simulink model "ex_modeling_components"  (R2020a)
settings: Solver=VariableStepAuto  StartTime=0.0  StopTime=10.0  RelTol=1e-3
libraries: simulink x1
settings Model: Creator=The MathWorks, Inc.  LastModifiedBy=Admin
settings DataIOCC: ReturnWorkspaceOutputs=off
settings DebuggingCC: PregeneratedLibrarySubsystemCodeDiagnostic=none  ArithmeticOperatorsInVariantConditions=warning
settings SFSimCC: SimUseLocalCustomCode=off  CustomCodeUndefinedFunction=UseInterfaceOnly
settings RTWCC: RTWUseLocalCustomCode=off

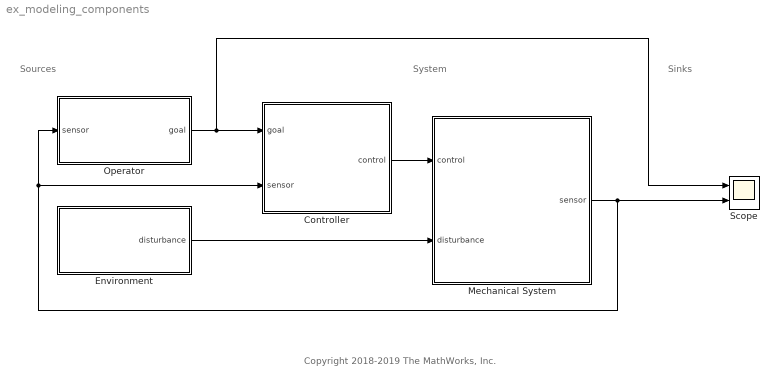
== system ex_modeling_components ==
  note: System
  note: Sources
  note: Copyright 2018-2019 The MathWorks, Inc.
  note: Sinks
  Controller : Subsystem  TreatAsAtomicUnit=on
  Environment : Subsystem
  Mechanical System : Subsystem
  Operator : Subsystem
  Scope : Scope  NumInputPorts=2
  wires:
  Controller/1(control) -> Mechanical System/1(control)
  Mechanical System/1(sensor) -> Operator/1(sensor), Controller/2(sensor), Scope/2
  Environment/1(disturbance) -> Mechanical System/2(disturbance)
  Operator/1(goal) -> Scope/1, Controller/1(goal)

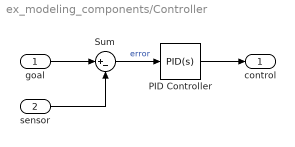
== system ex_modeling_components/Controller ==
  goal : Inport
  sensor : Inport  Port=2
  PID Controller : simulink/Continuous/PID Controller  Controller=PID  Form=Parallel  TimeDomain=Continuous-time  UseExternalTs=off  SampleTime=-1  IntegratorMethod=Forward Euler  FilterMethod=Forward Euler  ControllerParametersSource=internal  P=23.792676457344  I=17.7497318502065  D=7.56800739635058  UseFilter=on  N=49.2376691493838  TunerSelectOption=Transfer Function Based (PID Tuner App)  InitialConditionSource=internal  InitialConditionForIntegrator=0  InitialConditionForFilter=0  DifferentiatorICPrevScaledInput=0  ExternalReset=none  TrackingMode=off  Kt=1  LimitOutput=off  UpperSaturationLimit=inf  LowerSaturationLimit=-inf  LinearizeAsGain=on  AntiWindupMode=none  Kb=1  POutMin=[]  POutMax=[]  IOutMin=[]  IOutMax=[]  DOutMin=[]  DOutMax=[]  NOutMin=[]  NOutMax=[]  SumOutMin=[]  SumOutMax=[]  SaturationOutMin=[]  SaturationOutMax=[]  PParamMin=[]  PParamMax=[]  IParamMin=[]  IParamMax=[]  DParamMin=[]  DParamMax=[]  NParamMin=[]  NParamMax=[]  KbParamMin=[]  KbParamMax=[]  KtParamMin=[]  KtParamMax=[]  KbOutMin=[]  KbOutMax=[]  KtOutMin=[]  KtOutMax=[]  IntegratorOutMin=[]  IntegratorOutMax=[]  FilterOutMin=[]  FilterOutMax=[]  SumI1OutMin=[]  SumI1OutMax=[]  SumI2OutMin=[]  SumI2OutMax=[]  SumI3OutMin=[]  SumI3OutMax=[]  SumI4OutMin=[]  SumI4OutMax=[]  SumDOutMin=[]  SumDOutMax=[]  DifferentiatorOutMin=[]  DifferentiatorOutMax=[]  FilterDiffOutCoefMin=[]  FilterDiffOutCoefMax=[]  ReciprocalOutMin=[]  ReciprocalOutMax=[]  SumDenOutMin=[]  SumDenOutMax=[]  SumNumOutMin=[]  SumNumOutMax=[]  DivideOutMin=[]  DivideOutMax=[]  UdiffTsProdOutMin=[]  UdiffTsProdOutMax=[]  NTsProdOutMin=[]  NTsProdOutMax=[]  UintegralTsProdOutMin=[]  UintegralTsProdOutMax=[]  UngainTsProdOutMin=[]  UngainTsProdOutMax=[]  IntegratorContinuousStateAttributes=''  IntegratorStateMustResolveToSignalObject=off  IntegratorRTWStateStorageClass=Auto  FilterContinuousStateAttributes=''  FilterStateMustResolveToSignalObject=off  FilterRTWStateStorageClass=Auto  ParallelPVariant=InternalParameters  IdealPVariant=Disabled  IVariant=InternalParameters  DVariant=InternalParameters  IntegratorVariant=Continuous  SatVariant=Disabled  AWVariant=Passthrough  PCopyVariant=Disabled  TRVariant=Disabled  FdbkBlocksVariant=Forward  IdealPFdbkVariant=Disabled  SatFdbkVariant=Disabled  DerivativeFilterVariant=ContFilter  NVariant=InternalParameters  NCopyVariant=Disabled  FilterICVariant=InternalICsFilter  IntegratorICVariant=InternalICs  ExternalResetVariant=Disabled  TRSumVariant=Passthrough  SumFdbkVariant=Disabled  SumVariant=Sum_PID  TsampFilterVariant=InternalTs  TsampNgainVariant=Passthrough  TsampIntegralVariant=Passthrough
  Sum : Sum  Inputs=|+-
  control : Outport  VectorParamsAs1DForOutWhenUnconnected=off
  wires:
  goal/1 -> Sum/1
  Sum/1 -> PID Controller/1  "error"
  PID Controller/1 -> control/1
  sensor/1 -> Sum/2

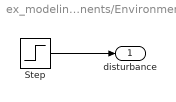
== system ex_modeling_components/Environment ==
  Step : Step  Time=5  After=10  SampleTime=0
  disturbance : Outport  VectorParamsAs1DForOutWhenUnconnected=off
  wires:
  Step/1 -> disturbance/1

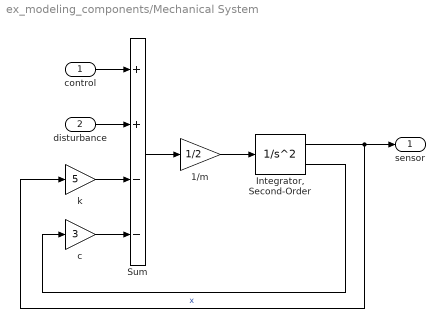
== system ex_modeling_components/Mechanical System ==
  control : Inport
  disturbance : Inport  Port=2
  1/m : Gain  Gain=1/2
  "Integrator, Second-Order" : SecondOrderIntegrator
  Sum : Sum  Inputs=++--
  c : Gain  Gain=3
  k : Gain  Gain=5
  sensor : Outport  VectorParamsAs1DForOutWhenUnconnected=off
  wires:
  "Integrator, Second-Order"/2 -> c/1
  c/1 -> Sum/4
  "Integrator, Second-Order"/1 -> sensor/1, k/1  "x"
  Sum/1 -> 1/m/1
  k/1 -> Sum/3
  1/m/1 -> "Integrator, Second-Order"/1
  control/1 -> Sum/1
  disturbance/1 -> Sum/2

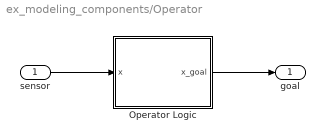
== system ex_modeling_components/Operator ==
  sensor : Inport
  Operator Logic : Stateflow chart  TreatAsAtomicUnit=on
  goal : Outport  VectorParamsAs1DForOutWhenUnconnected=off
  wires:
  sensor/1 -> Operator Logic/1(x)
  Operator Logic/1(x_goal) -> goal/1

== stateflow chart ex_modeling_components/Operator/Operator Logic ==
  state wait
    entry: x_goal = 0;
  state FirstOperation
    entry: x_goal = 2;
  state SecondOperation
    entry: x_goal = 1;
  wait -> FirstOperation : after(2,sec)
  FirstOperation -> SecondOperation : [x>2]
  (default) -> wait
  data: x input; x_goal output
